simulink model "sdrzWalkieTalkieTx"  (R2016a)
settings: Solver=ode45  StartTime=0.0  StopTime=inf  RelTol=1e-3
PostLoadFcn:
  | sdrzWalkieTalkieTxParams = sdrzWalkieTalkieTxHelper_SimParams();
  | sdrzWalkieTalkieTxHelper_ModelParamsMask('applyParametersToModel');
InitFcn:
  | sdrzWalkieTalkieTxParams = sdrzWalkieTalkieTxHelper_SimParams();
  | sdrzWalkieTalkieTxHelper_ModelParamsMask('applyParametersToModel');
libraries: dspsrcs4 x3, dspvision x1, sdrzblksprivate x1, sdrzlib x1, dspmlti4 x1
CloseFcn:
  | clear sdrzWalkieTalkieTxParams
Description:
  | This model uses Simulink(R) to transmit an FM signal suitable for reception on a commercial walkie-talkie using SDR hardware.
settings Model: SimulationMode=accelerator  Creator=The MathWorks, Inc.  LastModifiedBy=The MathWorks, Inc.
settings DataIOCC: LimitDataPoints=on  SaveFormat=Array
settings DebuggingCC: SolverPrmCheckMsg=warning  ParameterPrecisionLossMsg=none  AllowSymbolicDim=off
settings HardwareCC: ProdBitPerPointer=32  ProdLargestAtomicFloat=None  ProdIntDivRoundTo=Undefined  ProdEndianess=Unspecified  ProdWordSize=32  ProdHWDeviceType=32-bit Generic
settings ModelReferenceCC: PropagateSignalLabelsOutOfModel=off
settings ConfigComp: CovModelRefEnable=Off  CovSFcnEnable=off

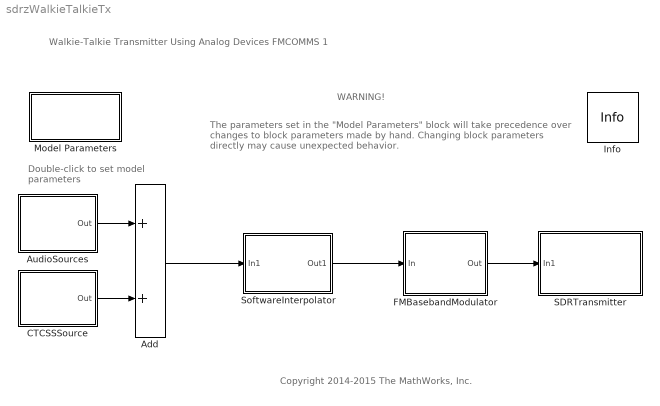
== system sdrzWalkieTalkieTx ==
  note: Walkie-Talkie Transmitter Using Analog Devices FMCOMMS 1
  note: Copyright 2014-2015 The MathWorks, Inc.
  note: Double-click to
      | set model parameters
  note: The parameters set in the "Model Parameters" block will
      | take precedence over changes to block parameters made by hand.
      | Changing block parameters directly may cause unexpected behavior.
  note: WARNING!
  Add : Sum
  AudioSources : Subsystem
      mask Display: fprintf('Audio\nGenerator');
  CTCSSSource : Subsystem
      mask Display: fprintf('CTCSS\nGenerator');
  FMBasebandModulator : Subsystem
      mask Display: disp('FM Baseband\nModulator');
  Info : sdrzblksprivate/Info  SystemSampleTime=-1
  Model Parameters : Subsystem  TreatAsAtomicUnit=on  SystemSampleTime=sdrzWalkieTalkieTxParams.audioSampleRate  mask(Model Parameters){audioSource=Sound file, toneFrequency=880, targetSweepTime=3, normalizedTransmitPower=0.9, walkieTalkieProtocol=FRS, channelFRS=1, channelPMR446=3, CTCSSCode=5, CTCSSAmplitude=0.15}
      mask prompts: audioSource "Signal selection:"; toneFrequency "Pure tone frequency (Hz):"; targetSweepTime "Chirp target/sweep time (s):"; normalizedTransmitPower "Normalized transmit power:"; walkieTalkieProtocol "Walkie-talkie protocol:"; channelFRS "Channel (1 to 14):"; channelPMR446 "Channel (1 to 8):"; CTCSSCode "CTCSS code (1 to 38):"; CTCSSAmplitude "Normalized CTCSS amplitude:"
      mask help: Changing these values defines the model parameters needed for a transmission.
      mask init:
      | sdrzWalkieTalkieTxHelper_ModelParamsMask('applyParametersToModel');
      mask Help: sdrzdemohelp;
      mask TypeOptions audioSource: Pure tone | Chirp | Sound file
      mask Callback audioSource: sdrzWalkieTalkieTxHelper_ModelParamsMask('maskDisplayUpdate');
      mask TypeOptions walkieTalkieProtocol: FRS | PMR446
      mask Callback walkieTalkieProtocol: sdrzWalkieTalkieTxHelper_ModelParamsMask('maskDisplayUpdate');
      mask Display: disp('Model\nParameters');
  SDRTransmitter : Subsystem
      mask Display: fprintf('SDR\nTransmitter')
  SoftwareInterpolator : Subsystem
      mask Display: fprintf('Software\nInterpolator')
  wires:
  CTCSSSource/1(Out) -> Add/2
  AudioSources/1(Out) -> Add/1
  Add/1 -> SoftwareInterpolator/1(In1)
  SoftwareInterpolator/1(Out1) -> FMBasebandModulator/1(In)
  FMBasebandModulator/1(Out) -> SDRTransmitter/1(In1)

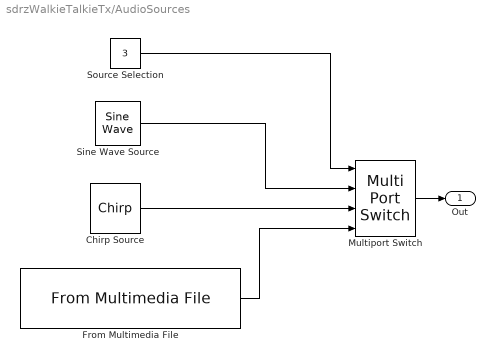
== system sdrzWalkieTalkieTx/AudioSources ==
  Chirp Source : dspsrcs4/Chirp  sweep=Linear  mode=Unidirectional  f0=500  f1=3400  t1=3  Tsweep=3  phase=0  Ts=sdrzWalkieTalkieTxParams.audioSamplePeriod  spf=sdrzWalkieTalkieTxParams.audioFrameSize  datatype=Single  OutputFrames=off
  From Multimedia File : dspvision/From Multimedia File  inputFilename=sdrzWalkieTalkieHelper_voice.wav  loop=on  numPlays=inf  outputStreams=Audio only  videoDataType=single  audioDataType=single  inheritSampleTime=on  userDefinedSampleTime=1/30  noAudioOutput=off  isIntensityVideo=off  fourcc=RGB  colorVideoFormat=Separate color signals  outputEOF=off  dataOrg=Column-major  audioFrameSize=sdrzWalkieTalkieTxParams.audioFrameSize  computeAudioFrameSize=off  outSamplingMode=Sample based
  Multiport Switch : MultiPortSwitch
  Sine Wave Source : dspsrcs4/Sine Wave  Amplitude=1  Frequency=880  Phase=0  SampleMode=Discrete  OutComplex=Real  CompMethod=Trigonometric fcn  TableSize=Speed  SampleTime=sdrzWalkieTalkieTxParams.audioSamplePeriod  SamplesPerFrame=sdrzWalkieTalkieTxParams.audioFrameSize  ResetState=Restart at time zero  OutputFrames=off  dataType=single  wordLen=16  udDataType=sfix(16)  fracBitsMode=Best precision  numFracBits=15  OutDataTypeStr=single  LastOutDataTypeStr=single
  Source Selection : Constant  Tag=SourceSelection  Value=3
  Out : Outport
  wires:
  Multiport Switch/1 -> Out/1
  Source Selection/1 -> Multiport Switch/1
  Chirp Source/1 -> Multiport Switch/3
  Sine Wave Source/1 -> Multiport Switch/2
  From Multimedia File/1 -> Multiport Switch/4

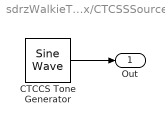
== system sdrzWalkieTalkieTx/CTCSSSource ==
  CTCCS Tone Generator : dspsrcs4/Sine Wave  Amplitude=0.15  Frequency=79.7  Phase=0  SampleMode=Discrete  OutComplex=Real  CompMethod=Trigonometric fcn  TableSize=Speed  SampleTime=sdrzWalkieTalkieTxParams.audioSamplePeriod  SamplesPerFrame=sdrzWalkieTalkieTxParams.audioFrameSize  ResetState=Restart at time zero  OutputFrames=off  dataType=single  wordLen=16  udDataType=sfix(16)  fracBitsMode=Best precision  numFracBits=15  OutDataTypeStr=single  LastOutDataTypeStr=single
  Out : Outport
  wires:
  CTCCS Tone Generator/1 -> Out/1

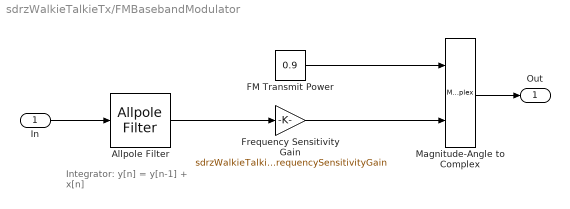
== system sdrzWalkieTalkieTx/FMBasebandModulator ==
  note: Integrator:
      | y[n] = y[n-1] + x[n]
  In : Inport
  Allpole Filter : AllpoleFilter  FilterStructure=Direct form transposed  Coefficients=[1 -1]  AccumDataTypeStr=Inherit: Same as product output  OutDataTypeStr=Inherit: Same as accumulator
  FM Transmit Power : Constant  Value=0.9  OutDataTypeStr=single
  Frequency Sensitivity Gain : Gain  Gain=sdrzWalkieTalkieTxParams.frequencySensitivityGain
  Magnitude-Angle to Complex : MagnitudeAngleToComplex
  Out : Outport
  wires:
  Frequency Sensitivity Gain/1 -> Magnitude-Angle to Complex/2
  Allpole Filter/1 -> Frequency Sensitivity Gain/1
  In/1 -> Allpole Filter/1
  Magnitude-Angle to Complex/1 -> Out/1
  FM Transmit Power/1 -> Magnitude-Angle to Complex/1

== system sdrzWalkieTalkieTx/Model Parameters ==
  note: This subsystem is empty.
      | It is used for setting parameter values (in the mask).

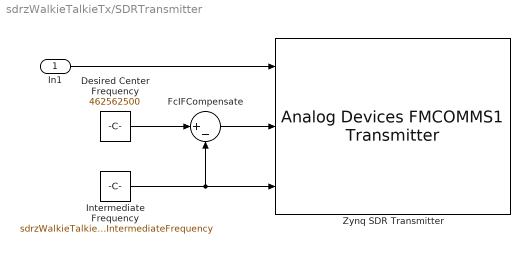
== system sdrzWalkieTalkieTx/SDRTransmitter ==
  In1 : Inport
  Desired Center Frequency : Constant  Value=462562500
  FcIFCompensate : Sum  Inputs=|+-
  Intermediate Frequency : Constant  Value=sdrzWalkieTalkieTxParams.radioIntermediateFrequency
  Zynq SDR Transmitter : sdrzlib/Analog Devices FMCOMMS1 Transmitter  SourceLibraryInfo="This block requires Communications System Toolbox Support Package for Xilinx FPGA-Based Radio. <a href=\"http://www.mathworks.com/hardware-support-packages\">More information</a>"  sobjType=comm.SDRZynqFMCOMMS1Transmitter  IPAddress=192.168.3.2  dataUDPPort=-1  ctrlUDPPort=-1  subDeviceList=comm.SDRZynqFMCOMMS1Transmitter  sdrBlockType=SDRBlockTypeSLT.SDRTxBlock  requester=UNUSED_BY_SFCN  sdrExecutionMode=HW  LostSamplesOutputPort=off  OutputDataType=int16  FrameLength=3660  EnableBurstMode=off  NumFramesInBurst=20  BypassUserLogic=on  InterpolatorSelect=DUC interpolator  SourceSelect=RF data  SineAmplitude=16000  SineFrequency=30000  EnableInternalClock=off  BypassIQBalance=off  CenterFrequencySource=Input port  CenterFrequency=467.6625e6 - 20e6  IntermediateFrequencySource=Input port  IntermediateFrequency=sdrzWalkieTalkieTxParams.radioIntermediateFrequency  IFBandwidthSource=Dialog  IFBandwidth=40e6  DACRateSource=Dialog  DACRate=sdrzWalkieTalkieTxParams.radioDACRate  GainSource=Dialog  Gain=4.5  InterpolationFactorSource=Dialog  InterpolationFactor=sdrzWalkieTalkieTxParams.radioInterpolationFactor  RFFrequencyIsTunable=logical(1)  SampleTime=0  BypassDCBlockingFilter=off  IQBalanceCoefficients=64  SkipAllHardwareResetAndInitialization=off  EnableIQCalibrationTable=on  CacheIQCalibrationTable=off
  wires:
  Intermediate Frequency/1 -> Zynq SDR Transmitter/3, FcIFCompensate/2
  Desired Center Frequency/1 -> FcIFCompensate/1
  FcIFCompensate/1 -> Zynq SDR Transmitter/2
  In1/1 -> Zynq SDR Transmitter/1

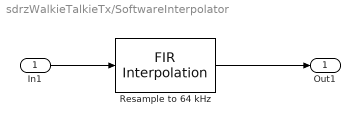
== system sdrzWalkieTalkieTx/SoftwareInterpolator ==
  In1 : Inport
  Resample to 64 kHz : dspmlti4/FIR Interpolation  FilterSource=Auto  h=sdrzWalkieTalkieTxParams.interpolatorCoefficients  L=sdrzWalkieTalkieTxParams.softwareInterpolationFactor  FilterObject=FINTERP  InputProcessing=Columns as channels (frame based)  framing=Enforce single-rate processing  outputBufInitCond=0  roundingMode=Floor  overflowMode=off  firstCoeffDataTypeStr=Inherit: Same word length as input  firstCoeffMin=[]  firstCoeffMax=[]  firstCoeffLastDataTypeStr=Inherit: Same word length as input  outputDataTypeStr=Inherit: Same as accumulator  outputMin=[]  outputMax=[]  outputLastDataTypeStr=Inherit: Same as accumulator
  Out1 : Outport
  wires:
  Resample to 64 kHz/1 -> Out1/1
  In1/1 -> Resample to 64 kHz/1
